simulink model "diagrama2B"  (Simulink 5.0)
settings: Solver=ode45  StartTime=0.0  StopTime=30000  RelTol=1e-3
libraries: simulink x4, dspstat3 x2, dsparch3 x1, dspmtrx3 x1, dspsigops x1
settings Model: LastModifiedBy=pc1

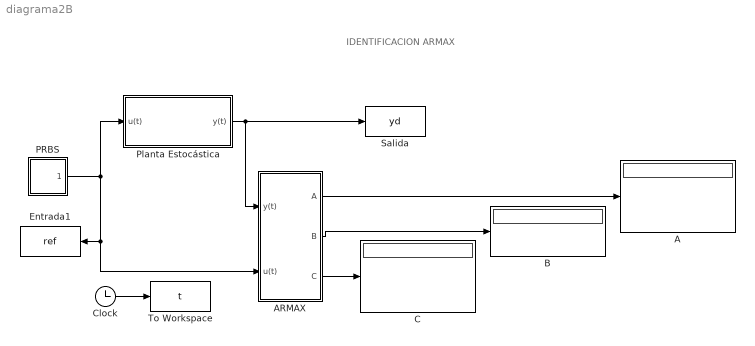
== system diagrama2B ==
  note: IDENTIFICACION ARMAX
  " PRBS" : Subsystem
  A : Display
  ARMAX : Subsystem
  B : Display
      settings: Format=bank
  C : Display
  Clock : Clock
      settings: Decimation=10
  Entrada1 : ToWorkspace  VariableName=ref  SampleTime=.1  SaveFormat=Array
  Planta Estocástica : Subsystem
  Salida : ToWorkspace  VariableName=yd  SampleTime=.1  SaveFormat=Array
  To Workspace : ToWorkspace  VariableName=t  SampleTime=.1  SaveFormat=Array
  wires:
  Clock/1 -> To Workspace/1
  ARMAX/2(B) -> B/1
  ARMAX/3(C) -> C/1
  Planta Estocástica/1(y(t)) -> Salida/1, ARMAX/1(y(t))
  " PRBS"/1(u ( t )) -> Planta Estocástica/1(u(t)), Entrada1/1, ARMAX/2(u(t))
  ARMAX/1(A) -> A/1

== system diagrama2B/ PRBS ==
  Random Number : RandomNumber  Variance=.001  SampleTime=0
  Sign : Signum
  Zero-Order Hold : ZeroOrderHold  SampleTime=.1
  u ( t ) : Outport
  wires:
  Zero-Order Hold/1 -> u ( t )/1
  Sign/1 -> Zero-Order Hold/1
  Random Number/1 -> Sign/1

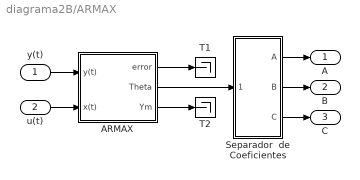
== system diagrama2B/ARMAX ==
  y(t) : Inport
  u(t) : Inport  Port=2
  ARMAX : Subsystem  mask{L=0.998, ts=.1, nk=0, na=3, nb=2, nc=3}
      mask prompts: L "valor landa"; ts "valor ts"; nk "valor nk"; na "Valor na"; nb "valor nb"; nc "valor nc"
  Separador  de Coeficientes : Subsystem  mask{na=3, nb=2, nc=3, ts=0.1}
      mask prompts: ts "Tiempo de Muestreo"
  T1 : Terminator
  T2 : Terminator
  A : Outport
  B : Outport  Port=2
  C : Outport  Port=3
  wires:
  Separador  de Coeficientes/3(C) -> C/1
  Separador  de Coeficientes/2(B) -> B/1
  Separador  de Coeficientes/1(A) -> A/1
  u(t)/1 -> ARMAX/2(x(t))
  y(t)/1 -> ARMAX/1(y(t))
  ARMAX/3(Ym) -> T2/1
  ARMAX/1(error) -> T1/1
  ARMAX/2(Theta) -> Separador  de Coeficientes/1(theta)

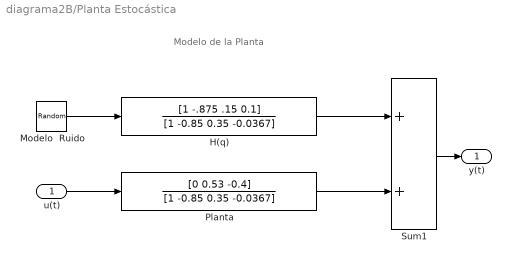
== system diagrama2B/Planta Estocástica ==
  note: Modelo de la Planta
  u(t) : Inport
  H(q) : DiscreteFilter  Numerator=[1 -.875 .15 0.1]  Denominator=[1 -0.85 0.35 -0.0367]  SampleTime=.1
  Modelo  Ruido : RandomNumber  Variance=.01  SampleTime=0.1
  Planta : DiscreteFilter  Numerator=[0 0.53 -0.4]  Denominator=[1 -0.85 0.35 -0.0367]  SampleTime=.1
  Sum1 : Sum  SaturateOnIntegerOverflow=on
  y(t) : Outport
  wires:
  Sum1/1 -> y(t)/1
  Planta/1 -> Sum1/2
  u(t)/1 -> Planta/1
  H(q)/1 -> Sum1/1
  Modelo  Ruido/1 -> H(q)/1

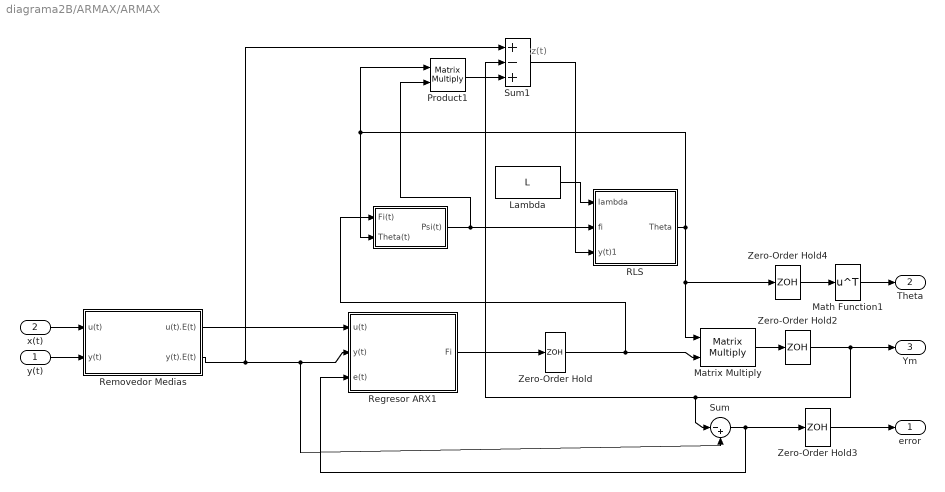
== system diagrama2B/ARMAX/ARMAX ==
  note: z(t)
  y(t) : Inport
  x(t) : Inport  Port=2
  "  " : Subsystem
  Lambda : Constant  Value=L  ShowAdditionalParam=on
  Math Function1 : Math  Operator=transpose
  Matrix Multiply : dspmtrx3/Matrix Multiply  numInputPorts=2  OptimizationLevel=None
  Product1 : Product  Multiplication=Matrix(*)  SaturateOnIntegerOverflow=on  InputSameDT=on
  RLS : Subsystem
  Regresor ARX1 : Subsystem
  Removedor Medias : Subsystem
  Sum : Sum  Inputs=|-+  SaturateOnIntegerOverflow=on  InputSameDT=on
  Sum1 : Sum  Inputs=+-+  SaturateOnIntegerOverflow=on  InputSameDT=on
  Zero-Order Hold{,2..4} (4 alike) : ZeroOrderHold  SampleTime=ts
  error : Outport
  Theta : Outport  Port=2
  Ym : Outport  Port=3
  wires:
  Math Function1/1 -> Theta/1
  Zero-Order Hold4/1 -> Math Function1/1
  RLS/1(Theta) -> Matrix Multiply/1, Zero-Order Hold4/1, "  "/2(Theta(t)), Product1/1
  Lambda/1 -> RLS/1(lambda)
  "  "/1(Psi(t)) -> RLS/2(fi), Product1/2
  Regresor ARX1/1(Fi) -> Zero-Order Hold/1
  Removedor Medias/2(y(t).E(t)) -> Sum/2, Regresor ARX1/2(y(t)), Sum1/1
  Removedor Medias/1(u(t).E(t)) -> Regresor ARX1/1(u(t))
  y(t)/1 -> Removedor Medias/2(y(t))
  x(t)/1 -> Removedor Medias/1(u(t))
  Zero-Order Hold/1 -> Matrix Multiply/2, "  "/1(Fi(t))
  Matrix Multiply/1 -> Zero-Order Hold2/1
  Zero-Order Hold2/1 -> Ym/1, Sum/1, Sum1/2
  Sum/1 -> Regresor ARX1/3(e(t)), Zero-Order Hold3/1
  Zero-Order Hold3/1 -> error/1
  Product1/1 -> Sum1/3
  Sum1/1 -> RLS/3(y(t)1)

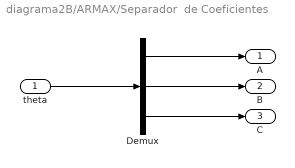
== system diagrama2B/ARMAX/Separador  de Coeficientes ==
  theta : Inport  PortDimensions=[na+nb+nc;1]  SampleTime=ts
  Demux : Demux  Outputs=[na,nb,nc]
  A : Outport
  B : Outport  Port=2
  C : Outport  Port=3
  wires:
  Demux/3 -> C/1
  Demux/2 -> B/1
  theta/1 -> Demux/1
  Demux/1 -> A/1

== system diagrama2B/ARMAX/ARMAX/   ==
  Fi(t) : Inport
  Theta(t) : Inport  Port=2
  filtro iir : Subsystem
  Psi(t) : Outport
  wires:
  filtro iir/1(Out1) -> Psi(t)/1
  Theta(t)/1 -> filtro iir/2(In2)
  Fi(t)/1 -> filtro iir/1(In1)

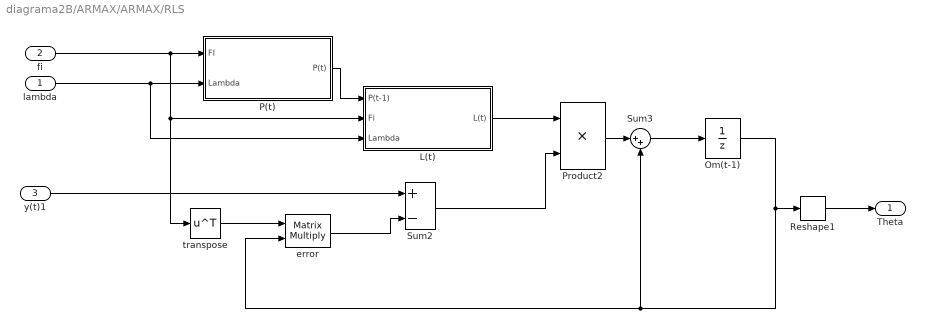
== system diagrama2B/ARMAX/ARMAX/RLS ==
  lambda : Inport
  fi : Inport  Port=2
  y(t)1 : Inport  Port=3
  L(t) : Subsystem
  Om(t-1) : UnitDelay  X0=zeros(1,na+nb+nc)'+.2  SampleTime=ts
  P(t) : Subsystem
  Product2 : Product  SaturateOnIntegerOverflow=on  InputSameDT=on
  Reshape1 : simulink/Math Operations/Reshape  OutputDimensionality=Row vector  OutputDimensions=[1,1]
  Sum2 : Sum  Inputs=+-  SaturateOnIntegerOverflow=on  InputSameDT=on
  Sum3 : Sum  Inputs=|++  SaturateOnIntegerOverflow=on  InputSameDT=on
  error : Product  Multiplication=Matrix(*)  SaturateOnIntegerOverflow=on  InputSameDT=on
  transpose : Math  Operator=transpose
  Theta : Outport
  wires:
  Reshape1/1 -> Theta/1
  lambda/1 -> L(t)/3(Lambda), P(t)/2(Lambda)
  fi/1 -> transpose/1, L(t)/2(Fi), P(t)/1(FI)
  P(t)/1("P(t) ") -> L(t)/1(P(t-1))
  L(t)/1(L(t)) -> Product2/1
  Product2/1 -> Sum3/1
  Sum3/1 -> Om(t-1)/1
  Sum2/1 -> Product2/2
  y(t)1/1 -> Sum2/1
  error/1 -> Sum2/2
  Om(t-1)/1 -> Reshape1/1, error/2, Sum3/2
  transpose/1 -> error/1

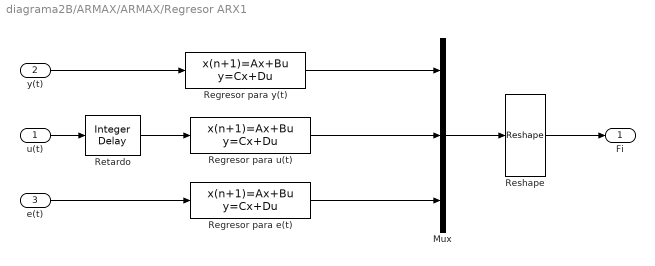
== system diagrama2B/ARMAX/ARMAX/Regresor ARX1 ==
  u(t) : Inport
  y(t) : Inport  Port=2
  e(t) : Inport  Port=3
  Mux : Mux  Inputs=3
  Regresor para e(t) : DiscreteStateSpace  A=[zeros(1,nc);eye(nc-1,nc)]  B=[1,zeros(1,nc-1)]'  C=eye(nc)  D=[zeros(nc,1)]  SampleTime=ts
  Regresor para u(t) : DiscreteStateSpace  A=[zeros(1,nb);eye(nb-1,nb)]  B=[1,zeros(1,nb-1)]'  C=eye(nb)  D=[zeros(nb,1)]  SampleTime=ts
  Regresor para y(t) : DiscreteStateSpace  A=[zeros(1,na);eye(na-1,na)]  B=[-1,zeros(1,na-1)]'  C=eye(na)  D=[zeros(na,1)]  SampleTime=ts
  Reshape : simulink/Math Operations/Reshape  OutputDimensionality=Column vector  OutputDimensions=[1,1]
  Retardo : dspsigops/Integer Delay  delay=nk  ic=0  reset_popup=None
  Fi : Outport
  wires:
  Regresor para e(t)/1 -> Mux/3
  Reshape/1 -> Fi/1
  Regresor para y(t)/1 -> Mux/1
  Regresor para u(t)/1 -> Mux/2
  y(t)/1 -> Regresor para y(t)/1
  Mux/1 -> Reshape/1
  u(t)/1 -> Retardo/1
  Retardo/1 -> Regresor para u(t)/1
  e(t)/1 -> Regresor para e(t)/1

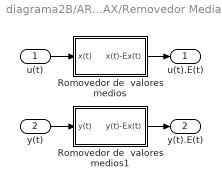
== system diagrama2B/ARMAX/ARMAX/Removedor Medias ==
  u(t) : Inport
  y(t) : Inport  Port=2
  Romovedor de  valores medios : Subsystem
  Romovedor de  valores medios1 : Subsystem
  u(t).E(t) : Outport
  y(t).E(t) : Outport  Port=2
  wires:
  Romovedor de  valores medios1/1(y(t)-Ex(t)) -> y(t).E(t)/1
  y(t)/1 -> Romovedor de  valores medios1/1(y(t))
  Romovedor de  valores medios/1(x(t)-Ex(t)) -> u(t).E(t)/1
  u(t)/1 -> Romovedor de  valores medios/1(x(t))

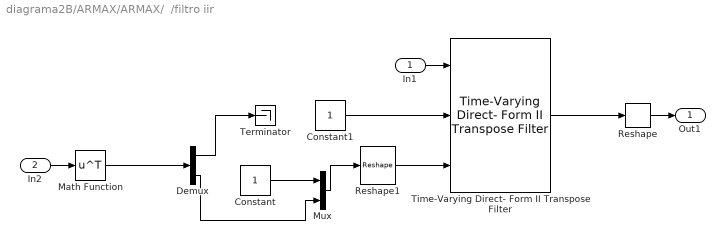
== system diagrama2B/ARMAX/ARMAX/  /filtro iir ==
  In1 : Inport
  In2 : Inport  Port=2
  Constant : Constant
  Constant1 : Constant
  Demux : Demux  Outputs=[na+nb,nc]
  Math Function : Math  Operator=transpose
  Mux : Mux  Inputs=2
  Reshape : simulink/Math Operations/Reshape  OutputDimensionality=Column vector  OutputDimensions=[1,1]
  Reshape1 : simulink/Math Operations/Reshape  OutputDimensionality=Column vector  OutputDimensions=[1,1]
  Terminator : Terminator
  Time-Varying Direct- Form II Transpose Filter : dsparch3/Time-Varying Direct- Form II Transpose Filter  NumDen=Pole-Zero (IIR)  ic=0  filtCheck=on  FiltPerFrame=One Filter Per Frame Time
  Out1 : Outport
  wires:
  In2/1 -> Math Function/1
  Reshape/1 -> Out1/1
  In1/1 -> Time-Varying Direct- Form II Transpose Filter/1
  Reshape1/1 -> Time-Varying Direct- Form II Transpose Filter/3
  Mux/1 -> Reshape1/1
  Math Function/1 -> Demux/1
  Demux/2 -> Mux/2
  Constant/1 -> Mux/1
  Constant1/1 -> Time-Varying Direct- Form II Transpose Filter/2
  Demux/1 -> Terminator/1
  Time-Varying Direct- Form II Transpose Filter/1 -> Reshape/1

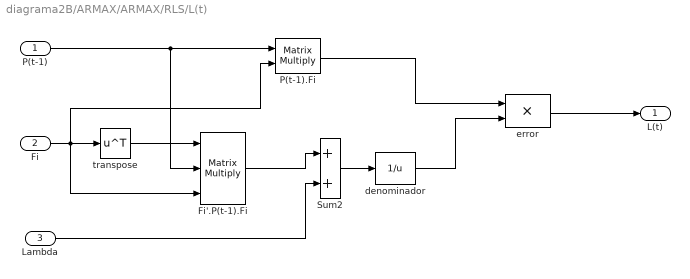
== system diagrama2B/ARMAX/ARMAX/RLS/L(t) ==
  P(t-1) : Inport
  Fi : Inport  Port=2
  Lambda : Inport  Port=3
  Fi'.P(t-1).Fi : Product  Inputs=3  Multiplication=Matrix(*)  SaturateOnIntegerOverflow=on  InputSameDT=on
  P(t-1).Fi : Product  Multiplication=Matrix(*)  ShowAdditionalParam=on  SaturateOnIntegerOverflow=on  InputSameDT=on
  Sum2 : Sum  ShowAdditionalParam=on  SaturateOnIntegerOverflow=on  InputSameDT=on
  denominador : Fcn  Expr=1/u
  error : Product  SaturateOnIntegerOverflow=on  InputSameDT=on
  transpose : Math  Operator=transpose
  L(t) : Outport
  wires:
  Lambda/1 -> Sum2/2
  Fi'.P(t-1).Fi/1 -> Sum2/1
  error/1 -> L(t)/1
  P(t-1)/1 -> P(t-1).Fi/1, Fi'.P(t-1).Fi/2
  P(t-1).Fi/1 -> error/1
  denominador/1 -> error/2
  Sum2/1 -> denominador/1
  transpose/1 -> Fi'.P(t-1).Fi/1
  Fi/1 -> Fi'.P(t-1).Fi/3, transpose/1, P(t-1).Fi/2

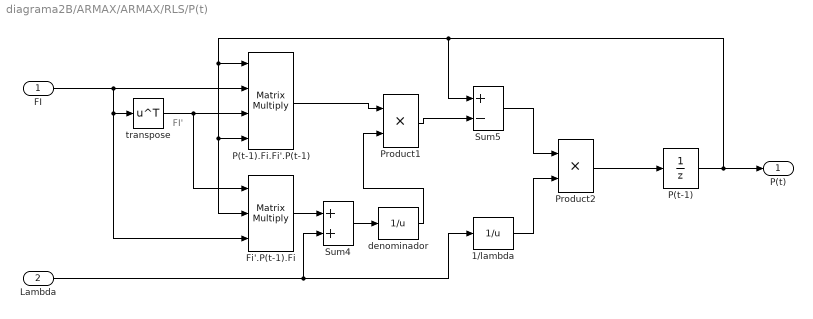
== system diagrama2B/ARMAX/ARMAX/RLS/P(t) ==
  note: FI'
  FI : Inport
  Lambda : Inport  Port=2
  1/lambda : Fcn  Expr=1/u
  Fi'.P(t-1).Fi : Product  Inputs=3  Multiplication=Matrix(*)  SaturateOnIntegerOverflow=on  InputSameDT=on
  P(t-1) : UnitDelay  X0=100000*eye(na+nb+nc)  SampleTime=ts
  P(t-1).Fi.Fi'.P(t-1) : Product  Inputs=4  Multiplication=Matrix(*)  SaturateOnIntegerOverflow=on  InputSameDT=on
  Product1 : Product  SaturateOnIntegerOverflow=on  InputSameDT=on
  Product2 : Product  SaturateOnIntegerOverflow=on  InputSameDT=on
  Sum4 : Sum  SaturateOnIntegerOverflow=on  InputSameDT=on
  Sum5 : Sum  Inputs=+-  SaturateOnIntegerOverflow=on  InputSameDT=on
  denominador : Fcn  Expr=1/u
  transpose : Math  Operator=transpose
  "P(t) " : Outport
  wires:
  denominador/1 -> Product1/2
  1/lambda/1 -> Product2/2
  Sum5/1 -> Product2/1
  Product1/1 -> Sum5/2
  P(t-1).Fi.Fi'.P(t-1)/1 -> Product1/1
  Sum4/1 -> denominador/1
  Fi'.P(t-1).Fi/1 -> Sum4/1
  P(t-1)/1 -> "P(t) "/1, Fi'.P(t-1).Fi/2, P(t-1).Fi.Fi'.P(t-1)/4, P(t-1).Fi.Fi'.P(t-1)/1, Sum5/1
  Product2/1 -> P(t-1)/1
  Lambda/1 -> Sum4/2, 1/lambda/1
  transpose/1 -> Fi'.P(t-1).Fi/1, P(t-1).Fi.Fi'.P(t-1)/3
  FI/1 -> P(t-1).Fi.Fi'.P(t-1)/2, transpose/1, Fi'.P(t-1).Fi/3

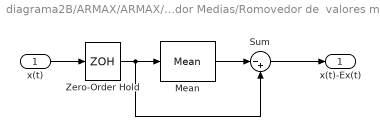
== system diagrama2B/ARMAX/ARMAX/Removedor Medias/Romovedor de  valores medios ==
  x(t) : Inport
  Mean : dspstat3/Mean  run=on  reset_popup=None
  Sum : Sum  Inputs=|-+  SaturateOnIntegerOverflow=on  InputSameDT=on
  Zero-Order Hold : ZeroOrderHold  SampleTime=ts
  x(t)-Ex(t) : Outport
  wires:
  Sum/1 -> x(t)-Ex(t)/1
  Mean/1 -> Sum/1
  Zero-Order Hold/1 -> Sum/2, Mean/1
  x(t)/1 -> Zero-Order Hold/1

== system diagrama2B/ARMAX/ARMAX/Removedor Medias/Romovedor de  valores medios1 ==
  y(t) : Inport
  Mean : dspstat3/Mean  run=on  reset_popup=None
  Sum : Sum  Inputs=|-+  SaturateOnIntegerOverflow=on  InputSameDT=on
  Zero-Order Hold : ZeroOrderHold  SampleTime=ts
  y(t)-Ex(t) : Outport
  wires:
  Sum/1 -> y(t)-Ex(t)/1
  Mean/1 -> Sum/1
  Zero-Order Hold/1 -> Sum/2, Mean/1
  y(t)/1 -> Zero-Order Hold/1
